simulink model "SimulationEnvManual"  (R2023b)
settings: Solver=VariableStepAuto  StartTime=0.0  StopTime=inf  RelTol=1e-3
undefined symbols (not defined in the file): act_mat, barometer, BIGL, drone, filter, imu, world
libraries: simulink x3, matrix_library x2, aerolibanimutils x2, vrlib x1, sim3dlib x1, uavsim3dlib x1
settings Model: Creator=HP  LastModifiedBy=jelho
settings OptimizationCC: ReuseModelBlockBuffer=off
settings DebuggingCC: AlgebraicLoopMsg=none

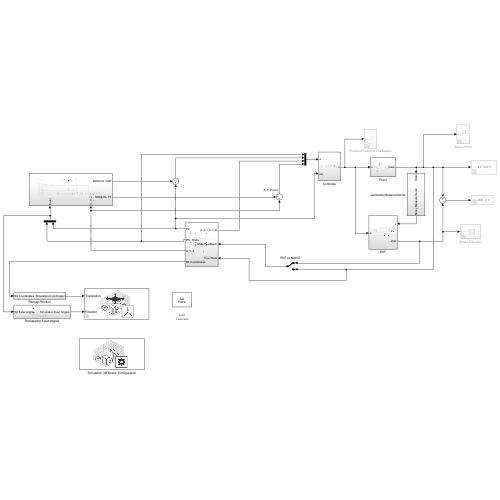
[thumbnail: Simulink's stored preview of the top-level diagram]
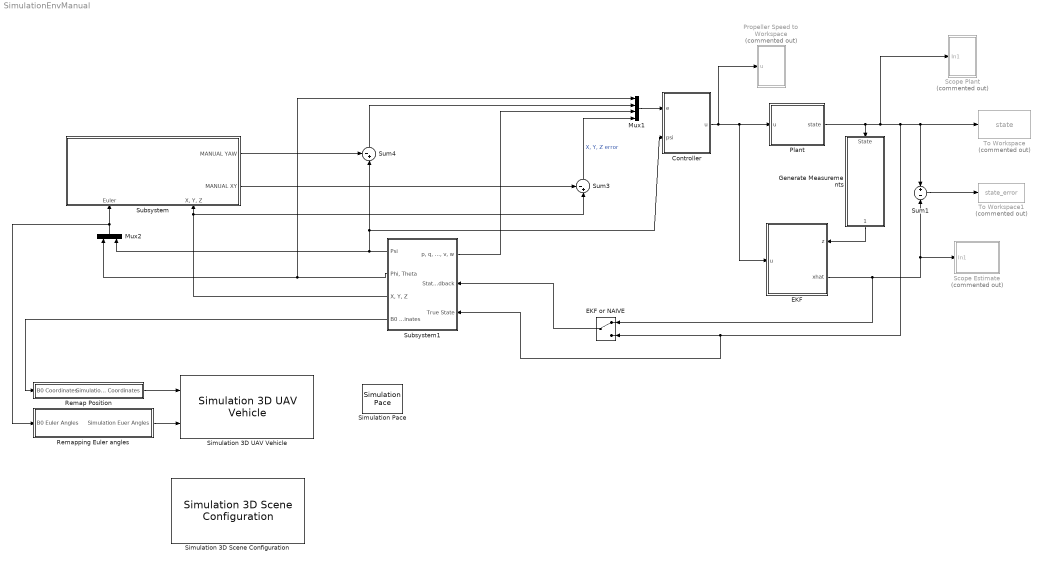
== system SimulationEnvManual ==
  Controller : Subsystem
  EKF : Subsystem
      settings: PortSchema="{\"entries\":[{\"content\":{\"sides\":[{\"content\":{\"connectorIds\":[\"In1\"]},\"type\":\"ConnectorPlacement.EquallySpacedRectSide\",\"uuid\":\"40613573-22c3-4397-8fb4-f3694734863a\"},{\"content\":{\"connectorIds\":[\"In2\",\"Out1\"],\"side\":\"RIGHT\"},\"type\":\"ConnectorPlacement.EquallySpacedRectSide\",\"uuid\":\"0d3695c7-8a5b-4700-a974-c5dffb14488a\"},{\"content\":{\"side\":\"TOP\"},\"type\":\"ConnectorPlacement.EquallySpacedRectSide\",\"uuid\":\"08eac33f-c286-45a0-82f1-214a32c22b76\"},{\"content\":{\"side\":\"BOTTOM\"},\"type\":\"ConnectorPlacement.EquallySpacedRectSide\",\"uuid\":\"51a49a93-d8bc-42ae-9bce-473bc1fc9d07\"}]},\"type\":\"ConnectorPlacement.EquallySpacedConnector\",\"uuid\":\"de3a0f79-73e9-4c25-bf5c-e7b3cc72a00c\"}],\"packageUris\":[\"http://schema.mathworks.com/mf0/Connector/R2020b\"],\"version\":\"1.0\"}"
  EKF or NAIVE : ManualSwitch
  Generate Measurements : Subsystem
  Mux1 : Mux
  Mux2 : Mux  Inputs=2
  Plant : Subsystem
  Propeller Speed to Workspace : Subsystem  Commented=on
  Remap Position : Subsystem
  Remapping Euler angles : Subsystem
  Scope Estimate : Subsystem  Commented=on
  Scope Plant : Subsystem  Commented=on
  Simulation 3D Scene Configuration : sim3dlib/Simulation 3D Scene Configuration  Priority=0  ProjectFormat=Default Scenes  SceneDesc=US city block  ProjectName=C:\Program Files\MATLAB\R2023b\toolbox\shared\sim3d_projects\automotive_project_windows\UE\WindowsNoEditor\VehicleSimulation.exe  ScenePath=/Game/Maps/USCityBlock  EnableOpenDRIVE=off  vehTagList={'Custom';'Scene Origin';'SimulinkVehicle1'}  vehTag=SimulinkVehicle1  FreeCameraInitialTranslation=[0, 0, 0]  FreeCameraDefaultInitialTranslation=[-6, 0, 2]  FreeCameraInitialRotation=[0, 0, 0]  FreeCameraDefaultInitialRotation=[0, -15, 0]  OpVisEn=off  Ts=1/60  EnableWindow=on  EnableRemoteAccess=off  EnableWeather=off  SunAltitude=40.0  SunAzimuth=90  clouds=10  wind=1  fog=0  rain=0  EnableGeospatial=off  OriginHeight=200  OriginLatitude=40.744652  OriginLongitude=-73.988864  MapStyle=Aerial  AdditionalAssetIDs=[]  UseAdvancedSunSky=off  SolarTime=11  TimeZone=-5  Day=21  Month=9  Year=2022  UseDaylightSavingTime=on  DSTStartDay=10  DSTStartMonth=3  DSTEndDay=3  DSTEndMonth=11  DSTSwitchHour=2  sensorTag=MainCamera1  sensorId=1  sensorName=MainCamera1  mountLoc=Origin  offsetFlag=off  tmountOffset=[0, 0, 0]  rmountOffset=[0, 0, 0]  HorizontalResolution=1280  VerticalResolution=720  HorizontalFOV=60  mountPoint=[0 0 0]  mountOrientation=[0 0 0]  aMode=4  ID=1  GeoTrigger=Inactive
      settings: LibrarySourceBlock=uavsim3dlib/Simulation 3D Scene Configuration
  Simulation 3D UAV Vehicle : uavsim3dlib/Simulation 3D UAV Vehicle  Priority=-1  Mesh=Quadrotor  MeshPath=/MathWorksUAVContent/UAVs/HexaRotorUAV/HexaRotor.HexaRotor  Color=Black  ActorName=SimulinkVehicle1  UseGlobalFrame=off  InitialTranslation=[0 0 0]  InitialRotation=[0 0 0]  InitialTranslationGlobal=[0 0 0]  InitialGeoOrigin=[0 0 0]  InitialRotationGlobal=[0 0 0]  SampleTime=-1  ActorType=SimulinkVehicle  ID=1  aMode=4  ActorTag=SimulinkVehicle1
  Simulation Pace : aerolibanimutils/Simulation Pace  SimulationPace=1  SleepMode=Auto  OutputPaceError=off  SampleTime=1/100
  Subsystem : Subsystem
      settings: PortSchema="{\"entries\":[{\"content\":{\"sides\":[{\"content\":{},\"type\":\"ConnectorPlacement.EquallySpacedRectSide\",\"uuid\":\"91d1624f-eb3c-4128-9ca0-0a39a1a4c695\"},{\"content\":{\"connectorIds\":[\"Out1\",\"Out2\"],\"side\":\"RIGHT\"},\"type\":\"ConnectorPlacement.EquallySpacedRectSide\",\"uuid\":\"1eacf8bd-a5e8-4d7e-b2c6-68202da0a464\"},{\"content\":{\"side\":\"TOP\"},\"type\":\"ConnectorPlacement.EquallySpacedRectSide\",\"uuid\":\"881c7496-1eb8-4ab1-ae56-46ea22276703\"},{\"content\":{\"connectorIds\":[\"In1\",\"In2\"],\"side\":\"BOTTOM\"},\"type\":\"ConnectorPlacement.EquallySpacedRectSide\",\"uuid\":\"54f45528-88dd-4514-ad9d-40f26d6e0713\"}]},\"type\":\"ConnectorPlacement.EquallySpacedConnector\",\"uuid\":\"c3aef092-554d-4415-a95e-e2ec15462ee3\"}],\"packageUris\":[\"http://schema.mathworks.com/mf0/Connector/R2020b\"],\"version\":\"1.0\"}"
  Subsystem1 : Subsystem
      settings: PortSchema="{\"entries\":[{\"content\":{\"sides\":[{\"content\":{\"connectorIds\":[\"Out2\",\"Out3\",\"Out4\",\"Out5\"]},\"type\":\"ConnectorPlacement.EquallySpacedRectSide\",\"uuid\":\"a354f8a1-719d-466d-a647-fe8a476dcf5d\"},{\"content\":{\"connectorIds\":[\"Out1\",\"In1\",\"In2\"],\"side\":\"RIGHT\"},\"type\":\"ConnectorPlacement.EquallySpacedRectSide\",\"uuid\":\"b9cb5ede-b59c-409e-8082-fb91c4f2361c\"},{\"content\":{\"side\":\"TOP\"},\"type\":\"ConnectorPlacement.EquallySpacedRectSide\",\"uuid\":\"8ee9585a-2649-44f5-b26b-06d86b499020\"}]},\"type\":\"ConnectorPlacement.EquallySpacedConnector\",\"uuid\":\"6c0311b6-aa0e-4aed-b018-d983f036a7c3\"}],\"packageUris\":[\"http://schema.mathworks.com/mf0/Connector/R2020b\"],\"version\":\"1.0\"}"
  Sum1 : Sum  Inputs=+-
  Sum3 : Sum  Inputs=-+|
  Sum4 : Sum  Inputs=-+|
  To Workspace : ToWorkspace  Commented=on  VariableName=state  SaveFormat=Timeseries  SampleTime=-1
  To Workspace1 : ToWorkspace  Commented=on  VariableName=state_error  SaveFormat=Timeseries  SampleTime=-1
  wires:
  Sum4/1 -> Mux1/2
  Controller/1(u) -> Plant/1(u), EKF/1(u), Propeller Speed to Workspace/1(u)
  Generate Measurements/1(Noisy Measurements) -> EKF/2(z)
  Sum1/1 -> To Workspace1/1
  Plant/1(state) -> Scope Plant/1(In1), Subsystem1/2(True State), EKF or NAIVE/2, To Workspace/1, Sum1/1, Generate Measurements/1(State)
  EKF/1(xhat) -> EKF or NAIVE/1, Sum1/2, Scope Estimate/1(In1)
  Subsystem1/1("p, q, r, u, v, w") -> Mux1/3
  Subsystem/1(MANUAL YAW) -> Sum4/1
  Sum3/1 -> Mux1/4  "X, Y, Z error"
  Subsystem/2(MANUAL XY) -> Sum3/1
  Subsystem1/3("Phi, Theta") -> Mux1/1, Mux2/1
  Subsystem1/2(Psi) -> Mux2/2, Sum4/2, Controller/2(psi)
  Mux2/1 -> Remapping Euler angles/1(B0 Euler Angles), Subsystem/1(Euler)
  Subsystem1/4("X, Y, Z") -> Sum3/2, Subsystem/2("X, Y, Z")
  Remapping Euler angles/1(Simulation Euer Angles) -> Simulation 3D UAV Vehicle/2
  Remap Position/1(Simulation Coordinates) -> Simulation 3D UAV Vehicle/1
  Mux1/1 -> Controller/1(e)
  EKF or NAIVE/1 -> Subsystem1/1(State Feedback)
  Subsystem1/5(B0 Coordinates) -> Remap Position/1(B0 Coordinates)

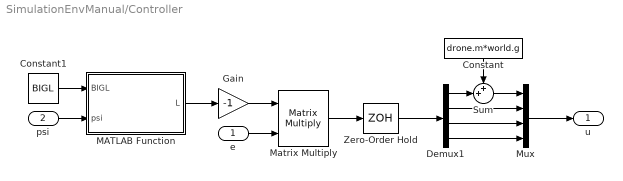
== system SimulationEnvManual/Controller ==
  e : Inport
  psi : Inport  Port=2
  Constant : Constant  Value=drone.m*world.g
  Constant1 : Constant  Value=BIGL
  Demux1 : Demux
  Gain : Gain  Gain=-1
  MATLAB Function : MATLAB Function  TreatAsAtomicUnit=on
  Matrix Multiply : Product  Multiplication=Matrix(*)
  Mux : Mux
  Sum : Sum  Inputs=++|
  Zero-Order Hold : ZeroOrderHold  SampleTime=0.01
  u : Outport
  wires:
  Demux1/3 -> Mux/3
  Demux1/2 -> Mux/2
  Mux/1 -> u/1
  Demux1/4 -> Mux/4
  Demux1/1 -> Sum/2
  Sum/1 -> Mux/1
  Constant/1 -> Sum/1
  Zero-Order Hold/1 -> Demux1/1
  e/1 -> Matrix Multiply/2
  Gain/1 -> Matrix Multiply/1
  Matrix Multiply/1 -> Zero-Order Hold/1
  MATLAB Function/1(L) -> Gain/1
  Constant1/1 -> MATLAB Function/1(BIGL)
  psi/1 -> MATLAB Function/2(psi)

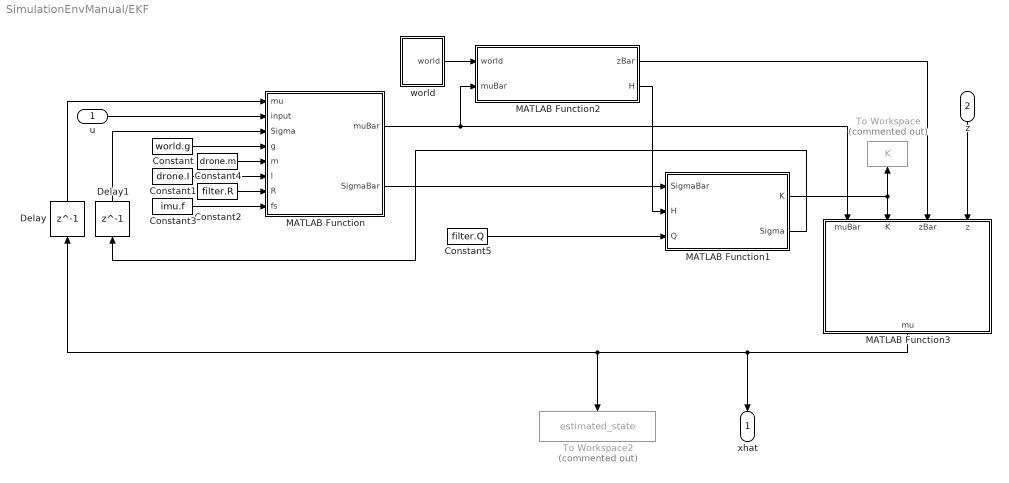
== system SimulationEnvManual/EKF ==
  u : Inport
  z : Inport  Port=2
  Constant : Constant  Value=world.g
  Constant1 : Constant  Value=drone.I
  Constant2 : Constant  Value=filter.R
  Constant3 : Constant  Value=imu.f
  Constant4 : Constant  Value=drone.m
  Constant5 : Constant  Value=filter.Q
  Delay : Delay  DelayLength=1  InitialCondition=filter.mu_0  SampleTime=0.01
  Delay1 : Delay  DelayLength=1  InitialCondition=filter.Sigma_0  SampleTime=0.01
  MATLAB Function : MATLAB Function  TreatAsAtomicUnit=on
  MATLAB Function1 : MATLAB Function  TreatAsAtomicUnit=on
  MATLAB Function2 : MATLAB Function  TreatAsAtomicUnit=on
  MATLAB Function3 : MATLAB Function  TreatAsAtomicUnit=on
  To Workspace : ToWorkspace  Commented=on  VariableName=K  SampleTime=-1
  To Workspace2 : ToWorkspace  Commented=on  VariableName=estimated_state  SaveFormat=Timeseries  SampleTime=-1
  world : Subsystem
  xhat : Outport
  wires:
  Constant2/1 -> MATLAB Function/7(R)
  MATLAB Function3/1(mu) -> Delay/1, To Workspace2/1, xhat/1
  MATLAB Function1/2(Sigma) -> Delay1/1
  MATLAB Function/1(muBar) -> MATLAB Function3/1(muBar), MATLAB Function2/2(muBar)
  Constant/1 -> MATLAB Function/4(g)
  MATLAB Function2/2(H) -> MATLAB Function1/2(H)
  Delay/1 -> MATLAB Function/1(mu)
  Constant1/1 -> MATLAB Function/6(I)
  MATLAB Function1/1(K) -> MATLAB Function3/2(K), To Workspace/1
  Constant5/1 -> MATLAB Function1/3(Q)
  MATLAB Function2/1(zBar) -> MATLAB Function3/3(zBar)
  Delay1/1 -> MATLAB Function/3(Sigma)
  Constant3/1 -> MATLAB Function/8(fs)
  Constant4/1 -> MATLAB Function/5(m)
  z/1 -> MATLAB Function3/4(z)
  MATLAB Function/2(SigmaBar) -> MATLAB Function1/1(SigmaBar)
  u/1 -> MATLAB Function/2(input)
  world/1(world) -> MATLAB Function2/1(world)

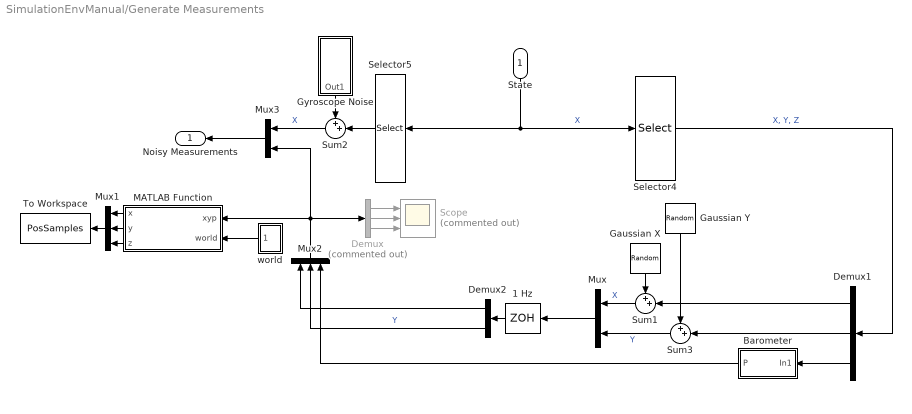
== system SimulationEnvManual/Generate Measurements ==
  State : Inport
  1 Hz : ZeroOrderHold
  Barometer : Subsystem
  Demux : Demux  Commented=on  Outputs=3
  Demux1 : Demux  Outputs=3
  Demux2 : Demux  Outputs=2
  Gaussian X : RandomNumber  Variance=4  Seed=[43121]  SampleTime=0.1
  Gaussian Y : RandomNumber  Variance=4  Seed=[43341]  SampleTime=0.1
  Gyroscope Noise : Subsystem
  MATLAB Function : MATLAB Function  TreatAsAtomicUnit=on
  Mux : Mux  Inputs=2
  Mux1 : Mux  Inputs=3
  Mux2 : Mux  Inputs=3
  Mux3 : Mux  Inputs=2
  Scope : Scope  Commented=on  NumInputPorts=3
  Selector4 : Selector  InputPortWidth=12  IndexOptions=Index vector (dialog)  Indices=[10 11 12]  OutputSizes=1
  Selector5 : Selector  InputPortWidth=12  IndexOptions=Index vector (dialog)  Indices=[1 2 3 4 5 6]  OutputSizes=1
  Sum1 : Sum  Inputs=++|
  Sum2 : Sum  Inputs=++|
  Sum3 : Sum  Inputs=++|
  To Workspace : ToWorkspace  VariableName=PosSamples  SaveFormat=Timeseries  SampleTime=-1
  world : Subsystem
  Noisy Measurements : Outport
  wires:
  Selector4/1 -> Demux1/1  "X, Y, Z"
  Mux2/1 -> Demux/1, Mux3/2, MATLAB Function/1(xyp)
  Demux2/1 -> Mux2/1
  1 Hz/1 -> Demux2/1
  Mux3/1 -> Noisy Measurements/1
  Mux/1 -> 1 Hz/1
  Demux2/2 -> Mux2/2  "Y"
  Gaussian X/1 -> Sum1/1
  Sum1/1 -> Mux/1  "X"
  Demux1/1 -> Sum1/2
  Sum3/1 -> Mux/2  "Y"
  Demux1/2 -> Sum3/2
  Gaussian Y/1 -> Sum3/1
  Demux/1 -> Scope/1
  Demux/2 -> Scope/2
  Demux/3 -> Scope/3
  Demux1/3 -> Barometer/1(In1)
  world/1(Out1) -> MATLAB Function/2(world)
  MATLAB Function/2(y) -> Mux1/2
  MATLAB Function/1(x) -> Mux1/1
  MATLAB Function/3(z) -> Mux1/3
  Mux1/1 -> To Workspace/1
  Selector5/1 -> Sum2/2
  Sum2/1 -> Mux3/1  "X"
  Gyroscope Noise/1(Out1) -> Sum2/1
  State/1 -> Selector5/1, Selector4/1  "X"
  Barometer/1(P) -> Mux2/3

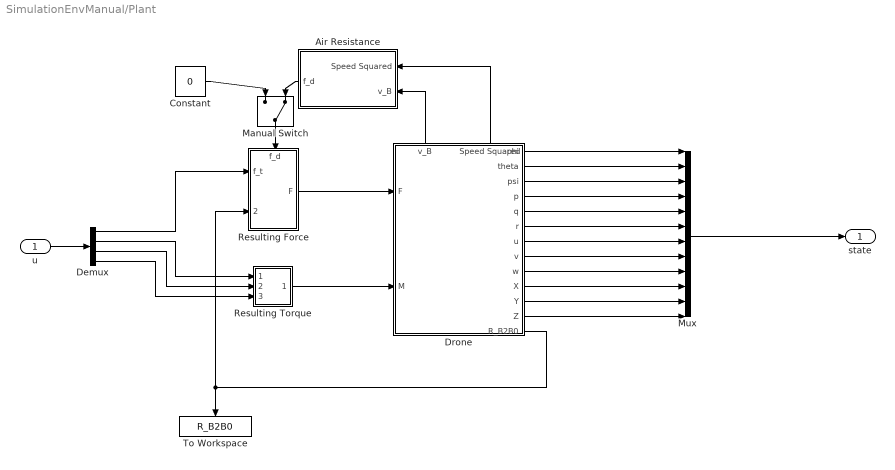
== system SimulationEnvManual/Plant ==
  u : Inport
  Air Resistance : Subsystem
  Constant : Constant  Value=0
  Demux : Demux
  Drone : Subsystem
      settings: PortSchema="{\"entries\":[{\"content\":{\"sides\":[{\"content\":{\"connectorIds\":[\"In1\",\"In2\"]},\"type\":\"ConnectorPlacement.EquallySpacedRectSide\",\"uuid\":\"8ffad7a2-32ec-43eb-87ee-fb2abc5db72d\"},{\"content\":{\"connectorIds\":[\"Out1\",\"Out2\",\"Out3\",\"Out4\",\"Out5\",\"Out6\",\"Out7\",\"Out8\",\"Out9\",\"Out10\",\"Out11\",\"Out12\",\"Out13\"],\"side\":\"RIGHT\"},\"type\":\"ConnectorPlacement.EquallySpacedRectSide\",\"uuid\":\"ca8d09d3-eea8-43a3-a12c-d896baab46a4\"},{\"content\":{\"connectorIds\":[\"Out14\",\"Out15\"],\"side\":\"TOP\"},\"type\":\"ConnectorPlacement.EquallySpacedRectSide\",\"uuid\":\"dfab79fc-8469-4116-b735-45bfaccfab37\"}]},\"type\":\"ConnectorPlacement.EquallySpacedConnector\",\"uuid\":\"bfc700f2-23fb-440c-b21c-b50295174d97\"}],\"packageUris\":[\"http://schema.mathworks.com/mf0/Connector/R2020b\"],\"version\":\"1.0\"}"
  Manual Switch : ManualSwitch  CurrentSetting=0
  Mux : Mux  Inputs=12
  Resulting Force : Subsystem
      settings: PortSchema="{\"entries\":[{\"content\":{\"sides\":[{\"content\":{\"connectorIds\":[\"In1\",\"In2\"]},\"type\":\"ConnectorPlacement.EquallySpacedRectSide\",\"uuid\":\"15f6bfea-ca78-407b-a070-46266de37f17\"},{\"content\":{\"connectorIds\":[\"Out1\"],\"side\":\"RIGHT\"},\"type\":\"ConnectorPlacement.EquallySpacedRectSide\",\"uuid\":\"1ac3e3a8-f699-47b6-93e9-6e96eb41779e\"},{\"content\":{\"connectorIds\":[\"In3\"],\"side\":\"TOP\"},\"type\":\"ConnectorPlacement.EquallySpacedRectSide\",\"uuid\":\"5f280c1d-1924-4695-afed-fbf3b3e218ac\"}]},\"type\":\"ConnectorPlacement.EquallySpacedConnector\",\"uuid\":\"fee2f4d4-3ff7-4dd2-b01a-205ded0d46ee\"}],\"packageUris\":[\"http://schema.mathworks.com/mf0/Connector/R2020b\"],\"version\":\"1.0\"}"
  Resulting Torque : Subsystem
  To Workspace : ToWorkspace  VariableName=R_B2B0  SampleTime=-1
  state : Outport
  wires:
  Drone/7(u) -> Mux/7
  Drone/2(theta) -> Mux/2
  Drone/4(p) -> Mux/4
  Drone/1(phi) -> Mux/1
  Drone/6(r) -> Mux/6
  Drone/9(w) -> Mux/9
  Resulting Torque/1(Out1) -> Drone/2(M)
  Drone/5(q) -> Mux/5
  Resulting Force/1(F) -> Drone/1(F)
  Drone/3(psi) -> Mux/3
  Drone/11(Y) -> Mux/11
  Drone/10(X) -> Mux/10
  Drone/8(v) -> Mux/8
  Drone/12(Z) -> Mux/12
  Drone/13(R_B2B0) -> Resulting Force/2(R_B2B0), To Workspace/1
  u/1 -> Demux/1
  Drone/14(v_B) -> Air Resistance/2(v_B)
  Drone/15(Speed Squared) -> Air Resistance/1(Speed Squared)
  Demux/1 -> Resulting Force/1(f_t)
  Demux/2 -> Resulting Torque/1(tau_x)
  Demux/3 -> Resulting Torque/2(tau_y)
  Demux/4 -> Resulting Torque/3(tau_z)
  Mux/1 -> state/1
  Manual Switch/1 -> Resulting Force/3(f_d)
  Air Resistance/1(f_d) -> Manual Switch/2
  Constant/1 -> Manual Switch/1

== system SimulationEnvManual/Propeller Speed to Workspace ==
  u : Inport
  Constant1 : Constant  Value=act_mat
  Matrix Multiply : Product  Multiplication=Matrix(*)
  To Workspace1 : ToWorkspace  VariableName=Input  SaveFormat=Timeseries  SampleTime=-1
  To Workspace2 : ToWorkspace  VariableName=PropSpeed  SaveFormat=Timeseries  SampleTime=-1
  wires:
  Matrix Multiply/1 -> To Workspace2/1
  u/1 -> Matrix Multiply/2, To Workspace1/1
  Constant1/1 -> Matrix Multiply/1

== system SimulationEnvManual/Remap Position ==
  B0 Coordinates : Inport
  Demux : Demux  Outputs=3
  Gain : Gain  Gain=-1
  Mux4 : Mux  Inputs=3
  Simulation Coordinates : Outport
  wires:
  Gain/1 -> Mux4/3
  Demux/1 -> Mux4/1
  B0 Coordinates/1 -> Demux/1
  Demux/3 -> Gain/1
  Mux4/1 -> Simulation Coordinates/1
  Demux/2 -> Mux4/2

== system SimulationEnvManual/Remapping Euler angles ==
  B0 Euler Angles : Inport
  Demux : Demux  Outputs=3
  Gain1 : Gain  Gain=-1
  Gain2 : Gain  Gain=-1
  Mux4 : Mux  Inputs=3
  Simulation Euer Angles : Outport
  wires:
  Demux/1 -> Gain2/1  "Roll"
  Demux/3 -> Mux4/1  "Yaw"
  Mux4/1 -> Simulation Euer Angles/1
  Demux/2 -> Gain1/1  "Pitch"
  B0 Euler Angles/1 -> Demux/1
  Gain1/1 -> Mux4/2
  Gain2/1 -> Mux4/3

== system SimulationEnvManual/Scope Estimate ==
  In1 : Inport
  Demux1 : Demux  Outputs=12
  Scope2 : Scope  NumInputPorts=12
  wires:
  Demux1/3 -> Scope2/3  "psi"
  Demux1/9 -> Scope2/9  "w"
  Demux1/10 -> Scope2/10  "X"
  Demux1/8 -> Scope2/8  "v"
  Demux1/5 -> Scope2/5  "q"
  Demux1/2 -> Scope2/2  "theta"
  Demux1/12 -> Scope2/12  "Z"
  Demux1/4 -> Scope2/4  "p"
  Demux1/6 -> Scope2/6  "r"
  Demux1/11 -> Scope2/11  "Y"
  Demux1/7 -> Scope2/7  "u"
  Demux1/1 -> Scope2/1  "phi"
  In1/1 -> Demux1/1

== system SimulationEnvManual/Scope Plant ==
  In1 : Inport
  Demux : Demux  Outputs=12
  Scope : Scope  NumInputPorts=12
  wires:
  Demux/9 -> Scope/9  "w"
  Demux/4 -> Scope/4  "p"
  Demux/12 -> Scope/12  "Z"
  Demux/2 -> Scope/2  "theta"
  Demux/6 -> Scope/6  "r"
  Demux/1 -> Scope/1  "phi"
  Demux/11 -> Scope/11  "Y"
  Demux/7 -> Scope/7  "u"
  Demux/10 -> Scope/10  "X"
  Demux/8 -> Scope/8  "v"
  Demux/3 -> Scope/3  "psi"
  Demux/5 -> Scope/5  "q"
  In1/1 -> Demux/1

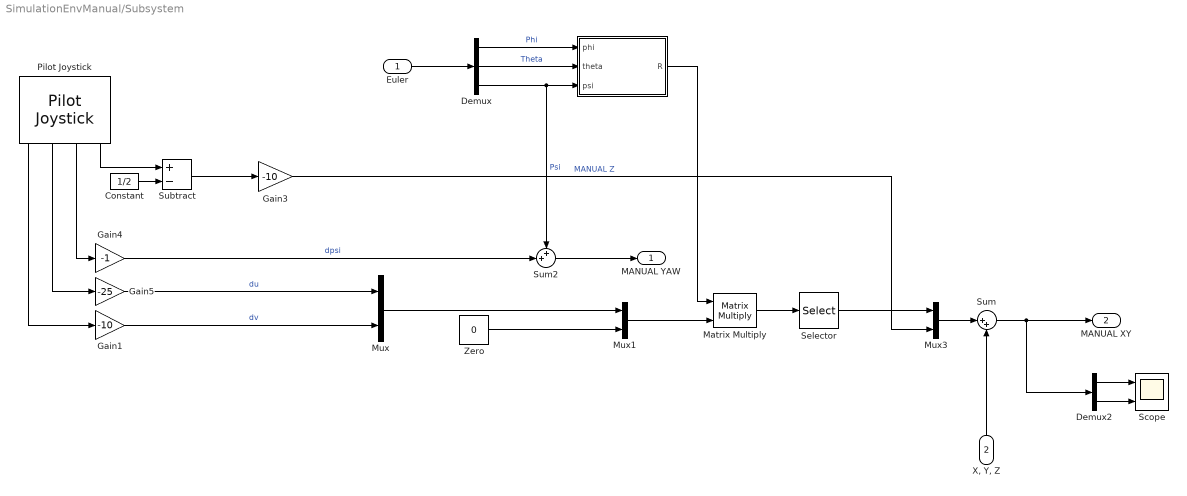
== system SimulationEnvManual/Subsystem ==
  Euler : Inport
  "X, Y, Z" : Inport  Port=2
  " " : MATLAB Function  TreatAsAtomicUnit=on
  Constant : Constant  Value=1/2
  Demux : Demux  Outputs=3
  Demux2 : Demux  Outputs=2
  Gain1 : Gain  Gain=-10
  Gain3 : Gain  Gain=-10
  Gain4 : Gain  Gain=-1
  Gain5 : Gain  Gain=-25
  Matrix Multiply : Product  Multiplication=Matrix(*)
  Mux : Mux  Inputs=2
  Mux1 : Mux  Inputs=2
  Mux3 : Mux  Inputs=2
  Pilot Joystick : aerolibanimutils/Pilot Joystick  JoystickID=Joystick1  OutputConfiguration=FourAxis  SampleTime=1/30
  Scope : Scope  NumInputPorts=2
  Selector : Selector  InputPortWidth=3  IndexOptions=Index vector (dialog)  Indices=[1 2]  OutputSizes=1
  Subtract : Sum  Inputs=+-
  Sum : Sum  Inputs=|++
  Sum2 : Sum  Inputs=++|
  Zero : Constant  Value=0  OutDataTypeStr=Inherit: Inherit via back propagation
  MANUAL YAW : Outport
  MANUAL XY : Outport  Port=2
  wires:
  Pilot Joystick/2 -> Gain5/1
  Pilot Joystick/3 -> Gain4/1
  Gain4/1 -> Sum2/2  "dpsi"
  Pilot Joystick/1 -> Gain1/1
  Pilot Joystick/4 -> Subtract/1
  Constant/1 -> Subtract/2
  Subtract/1 -> Gain3/1
  Gain3/1 -> Mux3/2  "MANUAL Z"
  Mux/1 -> Mux1/1
  Gain5/1 -> Mux/1  "du"
  Gain1/1 -> Mux/2  "dv"
  Euler/1 -> Demux/1
  Demux/1 -> " "/1(phi)  "Phi"
  Demux/2 -> " "/2(theta)  "Theta"
  Demux/3 -> " "/3(psi), Sum2/1  "Psi"
  Zero/1 -> Mux1/2
  Mux1/1 -> Matrix Multiply/2
  " "/1(R) -> Matrix Multiply/1
  Matrix Multiply/1 -> Selector/1
  Selector/1 -> Mux3/1
  "X, Y, Z"/1 -> Sum/2
  Sum/1 -> MANUAL XY/1, Demux2/1
  Sum2/1 -> MANUAL YAW/1
  Demux2/1 -> Scope/1
  Demux2/2 -> Scope/2
  Mux3/1 -> Sum/1

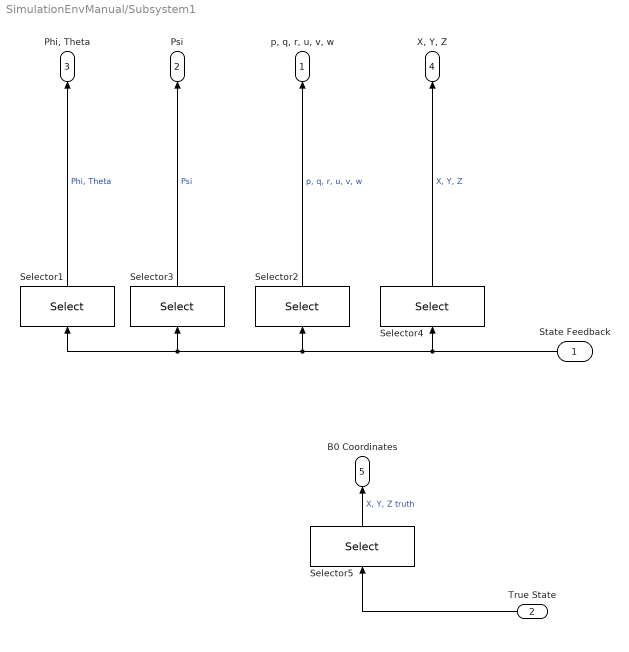
== system SimulationEnvManual/Subsystem1 ==
  State Feedback : Inport
  True State : Inport  Port=2
  Selector1 : Selector  InputPortWidth=12  IndexOptions=Index vector (dialog)  Indices=[1 2]  OutputSizes=1
  Selector2 : Selector  InputPortWidth=12  IndexOptions=Index vector (dialog)  Indices=[4 5 6 7 8 9]  OutputSizes=1
  Selector3 : Selector  InputPortWidth=12  IndexOptions=Index vector (dialog)  Indices=[3]  OutputSizes=1
  Selector4 : Selector  InputPortWidth=12  IndexOptions=Index vector (dialog)  Indices=[10 11 12]  OutputSizes=1
  Selector5 : Selector  InputPortWidth=12  IndexOptions=Index vector (dialog)  Indices=[10 11 12]  OutputSizes=1
  "p, q, r, u, v, w" : Outport
  Psi : Outport  Port=2
  "Phi, Theta" : Outport  Port=3
  "X, Y, Z" : Outport  Port=4
  B0 Coordinates : Outport  Port=5
  wires:
  Selector3/1 -> Psi/1  "Psi"
  Selector4/1 -> "X, Y, Z"/1  "X, Y, Z"
  State Feedback/1 -> Selector4/1, Selector1/1, Selector3/1, Selector2/1
  Selector1/1 -> "Phi, Theta"/1  "Phi, Theta"
  Selector2/1 -> "p, q, r, u, v, w"/1  "p, q, r, u, v, w"
  True State/1 -> Selector5/1
  Selector5/1 -> B0 Coordinates/1  "X, Y, Z truth"

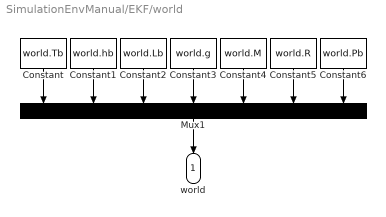
== system SimulationEnvManual/EKF/world ==
  Constant : Constant  Value=world.Tb
  Constant1 : Constant  Value=world.hb
  Constant2 : Constant  Value=world.Lb
  Constant3 : Constant  Value=world.g
  Constant4 : Constant  Value=world.M
  Constant5 : Constant  Value=world.R
  Constant6 : Constant  Value=world.Pb
  Mux1 : Mux  Inputs=7
  world : Outport
  wires:
  Constant2/1 -> Mux1/3
  Mux1/1 -> world/1
  Constant4/1 -> Mux1/5
  Constant3/1 -> Mux1/4
  Constant5/1 -> Mux1/6
  Constant/1 -> Mux1/1
  Constant1/1 -> Mux1/2
  Constant6/1 -> Mux1/7

== system SimulationEnvManual/Generate Measurements/Barometer ==
  In1 : Inport
  10 Hz : ZeroOrderHold  SampleTime=0.1
  Constant : Constant  Value=barometer.std
  MATLAB Function : MATLAB Function  TreatAsAtomicUnit=on
  world : Subsystem
  P : Outport
  wires:
  In1/1 -> 10 Hz/1
  10 Hz/1 -> MATLAB Function/1(Z)
  Constant/1 -> MATLAB Function/2(std)
  MATLAB Function/1(P) -> P/1  "P"
  world/1(Out1) -> MATLAB Function/3(world)

== system SimulationEnvManual/Generate Measurements/Gyroscope Noise ==
  " Phi" : RandomNumber  Variance=[((pi/180))^2]  Seed=[43341]  SampleTime=0.01
  " Psi" : RandomNumber  Variance=[((pi/180))^2]  Seed=[43751]  SampleTime=0.01
  " Theta" : RandomNumber  Variance=[((pi/180))^2]  Seed=[47341]  SampleTime=0.01
  " p" : RandomNumber  Variance=[((pi/180)*2.5)^2]  Seed=[41341]  SampleTime=0.01
  " q" : RandomNumber  Variance=[((pi/180)*2.5)^2]  Seed=[43631]  SampleTime=0.01
  " r" : RandomNumber  Variance=[((pi/180)*2.5)^2]  Seed=[67842]  SampleTime=0.01
  Mux4 : Mux  Inputs=6
  Out1 : Outport
  wires:
  " r"/1 -> Mux4/6
  " q"/1 -> Mux4/5
  Mux4/1 -> Out1/1
  " p"/1 -> Mux4/4
  " Phi"/1 -> Mux4/1
  " Theta"/1 -> Mux4/2
  " Psi"/1 -> Mux4/3

== system SimulationEnvManual/Generate Measurements/world ==
  Constant : Constant  Value=world.Tb
  Constant1 : Constant  Value=world.hb
  Constant2 : Constant  Value=world.Lb
  Constant3 : Constant  Value=world.g
  Constant4 : Constant  Value=world.M
  Constant5 : Constant  Value=world.R
  Constant6 : Constant  Value=world.Pb
  Mux1 : Mux  Inputs=7
  Out1 : Outport
  wires:
  Constant2/1 -> Mux1/3
  Mux1/1 -> Out1/1
  Constant4/1 -> Mux1/5
  Constant3/1 -> Mux1/4
  Constant5/1 -> Mux1/6
  Constant/1 -> Mux1/1
  Constant1/1 -> Mux1/2
  Constant6/1 -> Mux1/7

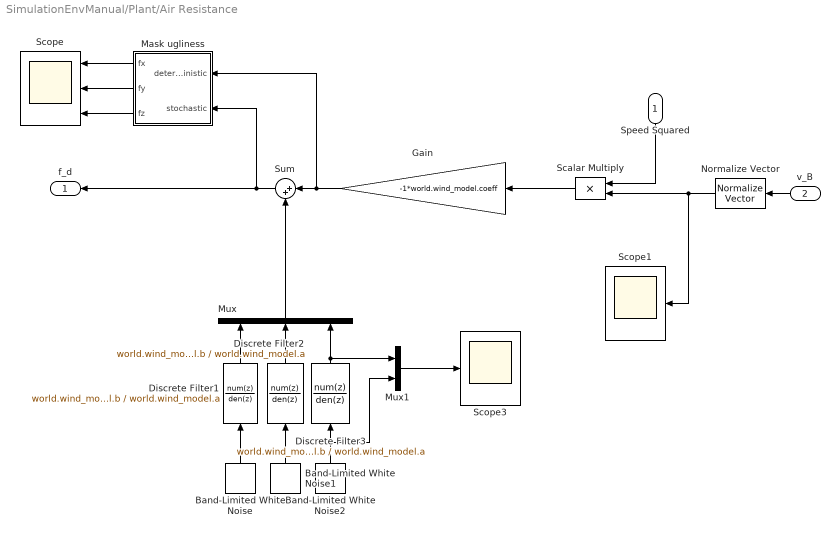
== system SimulationEnvManual/Plant/Air Resistance ==
  Speed Squared : Inport
  v_B : Inport  Port=2
  Band-Limited White Noise : simulink/Sources/Band-Limited White Noise  Cov=[0.001]  Ts=0.01  seed=[23351]
  Band-Limited White Noise1 : simulink/Sources/Band-Limited White Noise  Cov=[0.001]  Ts=0.01  seed=[23341]
  Band-Limited White Noise2 : simulink/Sources/Band-Limited White Noise  Cov=[0.001]  Ts=0.01  seed=[86328]
  Discrete Filter1 : DiscreteFilter  Numerator=world.wind_model.b  Denominator=world.wind_model.a
  Discrete Filter2 : DiscreteFilter  Numerator=world.wind_model.b  Denominator=world.wind_model.a
  Discrete Filter3 : DiscreteFilter  Numerator=world.wind_model.b  Denominator=world.wind_model.a
  Gain : Gain  Gain=-1*world.wind_model.coeff
  Mask ugliness : Subsystem
  Mux : Mux  Inputs=3
  Mux1 : Mux  Inputs=2
  Normalize Vector : vrlib/Utilities/Normalize Vector  maxzero=0
  Scalar Multiply : Product
  Scope : Scope  NumInputPorts=3
  Scope1 : Scope
  Scope3 : Scope
  Sum : Sum  Inputs=|++
  f_d : Outport
  wires:
  Normalize Vector/1 -> Scope1/1, Scalar Multiply/2
  Band-Limited White Noise/1 -> Discrete Filter1/1
  Band-Limited White Noise2/1 -> Mux1/2, Discrete Filter3/1
  Mux/1 -> Sum/2
  Gain/1 -> Mask ugliness/1(deterministic), Sum/1
  Sum/1 -> Mask ugliness/2(stochastic), f_d/1
  Mask ugliness/1(fx) -> Scope/1
  Mask ugliness/2(fy) -> Scope/2
  Mask ugliness/3(fz) -> Scope/3
  Discrete Filter1/1 -> Mux/1
  Discrete Filter2/1 -> Mux/2
  Discrete Filter3/1 -> Mux/3, Mux1/1
  v_B/1 -> Normalize Vector/1
  Scalar Multiply/1 -> Gain/1
  Speed Squared/1 -> Scalar Multiply/1
  Mux1/1 -> Scope3/1
  Band-Limited White Noise1/1 -> Discrete Filter2/1

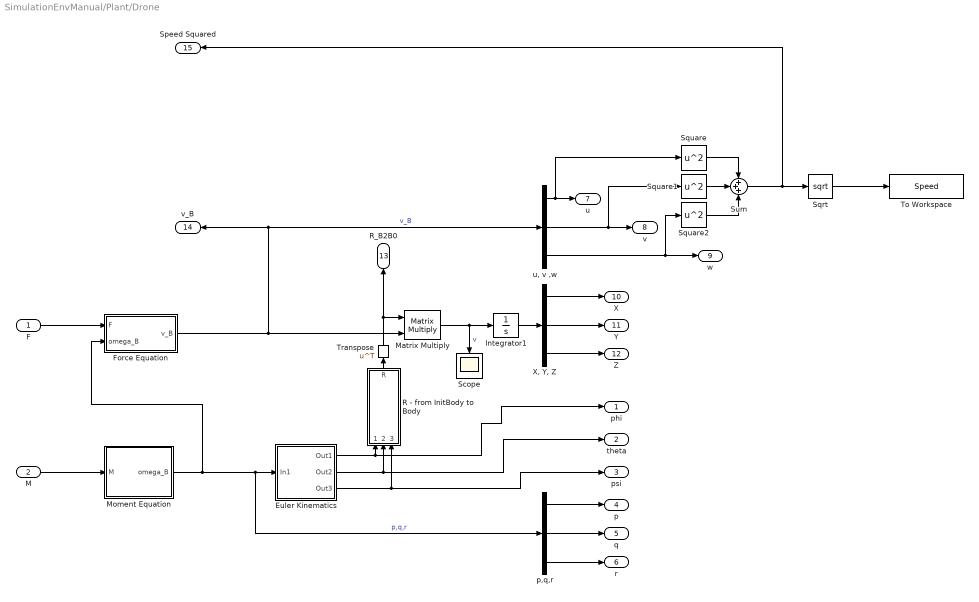
== system SimulationEnvManual/Plant/Drone ==
  F : Inport
  M : Inport  Port=2
  Euler Kinematics : Subsystem
  Force Equation : Subsystem
  Integrator1 : Integrator  InitialCondition=[0,0,0]
  Matrix Multiply : Product  Multiplication=Matrix(*)
  Moment Equation : Subsystem
  R - from InitBody to Body : MATLAB Function  TreatAsAtomicUnit=on
  Scope : Scope
  Sqrt : Sqrt
  Square : Math  Operator=square
  Square1 : Math  Operator=square
  Square2 : Math  Operator=square
  Sum : Sum  Inputs=+++
  To Workspace : ToWorkspace  VariableName=Speed  SaveFormat=Timeseries  SampleTime=-1
  Transpose : Math  Operator=transpose
  "X, Y, Z" : Demux  Outputs=3
  p,q,r : Demux  Outputs=3
  "u, v ,w" : Demux  Outputs=3
  phi : Outport
  theta : Outport  Port=2
  psi : Outport  Port=3
  p : Outport  Port=4
  q : Outport  Port=5
  r : Outport  Port=6
  u : Outport  Port=7
  v : Outport  Port=8
  w : Outport  Port=9
  X : Outport  Port=10
  Y : Outport  Port=11
  Z : Outport  Port=12
  R_B2B0 : Outport  Port=13
  v_B : Outport  Port=14
  Speed Squared : Outport  Port=15
  wires:
  Force Equation/1(v_B) -> Matrix Multiply/2, "u, v ,w"/1, v_B/1  "v_B"
  Euler Kinematics/2(Out2) -> R - from InitBody to Body/2(theta), theta/1
  Euler Kinematics/3(Out3) -> psi/1, R - from InitBody to Body/3(psi)
  "u, v ,w"/2 -> Square1/1, v/1
  "X, Y, Z"/1 -> X/1
  Integrator1/1 -> "X, Y, Z"/1
  Moment Equation/1(omega_B) -> p,q,r/1, Euler Kinematics/1(In1), Force Equation/2(omega_B)  "p,q,r"
  Euler Kinematics/1(Out1) -> R - from InitBody to Body/1(phi), phi/1
  "X, Y, Z"/2 -> Y/1
  Matrix Multiply/1 -> Integrator1/1, Scope/1  "v"
  F/1 -> Force Equation/1(F)
  "X, Y, Z"/3 -> Z/1
  M/1 -> Moment Equation/1(M)
  "u, v ,w"/3 -> Square2/1, w/1
  "u, v ,w"/1 -> Square/1, u/1
  p,q,r/2 -> q/1
  p,q,r/1 -> p/1
  p,q,r/3 -> r/1
  R - from InitBody to Body/1(R) -> Transpose/1
  Transpose/1 -> Matrix Multiply/1, R_B2B0/1
  Square/1 -> Sum/1
  Square1/1 -> Sum/2
  Square2/1 -> Sum/3
  Sum/1 -> Speed Squared/1, Sqrt/1
  Sqrt/1 -> To Workspace/1

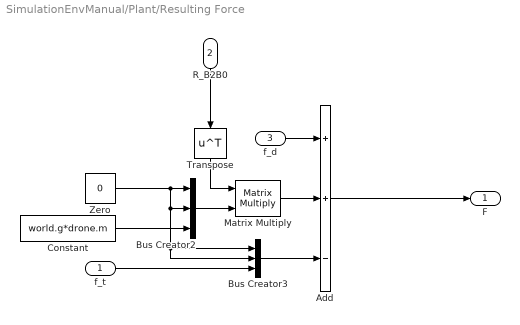
== system SimulationEnvManual/Plant/Resulting Force ==
  f_t : Inport
  R_B2B0 : Inport  Port=2
  f_d : Inport  Port=3
  Add : Sum  Inputs=++-
  Bus Creator2 : BusCreator  Inputs=3
  Bus Creator3 : BusCreator  Inputs=3
  Constant : Constant  Value=world.g*drone.m
  Matrix Multiply : Product  Multiplication=Matrix(*)
  Transpose : Math  Operator=transpose
  Zero : Constant  Value=0  OutDataTypeStr=Inherit: Inherit via back propagation
  F : Outport
  wires:
  Matrix Multiply/1 -> Add/2
  Bus Creator2/1 -> Matrix Multiply/2
  Add/1 -> F/1
  Zero/1 -> Bus Creator2/2, Bus Creator3/1, Bus Creator3/2, Bus Creator2/1
  R_B2B0/1 -> Transpose/1
  Constant/1 -> Bus Creator2/3
  Transpose/1 -> Matrix Multiply/1
  f_t/1 -> Bus Creator3/3
  Bus Creator3/1 -> Add/3
  f_d/1 -> Add/1

== system SimulationEnvManual/Plant/Resulting Torque ==
  tau_x : Inport
  tau_y : Inport  Port=2
  tau_z : Inport  Port=3
  Bus Creator2 : BusCreator  Inputs=3
  Out1 : Outport
  wires:
  tau_z/1 -> Bus Creator2/3
  Bus Creator2/1 -> Out1/1
  tau_x/1 -> Bus Creator2/1
  tau_y/1 -> Bus Creator2/2

== system SimulationEnvManual/Generate Measurements/Barometer/world ==
  Constant : Constant  Value=world.Tb
  Constant1 : Constant  Value=world.hb
  Constant2 : Constant  Value=world.Lb
  Constant3 : Constant  Value=world.g
  Constant4 : Constant  Value=world.M
  Constant5 : Constant  Value=world.R
  Constant6 : Constant  Value=world.Pb
  Mux1 : Mux  Inputs=7
  Out1 : Outport
  wires:
  Constant2/1 -> Mux1/3
  Mux1/1 -> Out1/1
  Constant4/1 -> Mux1/5
  Constant3/1 -> Mux1/4
  Constant5/1 -> Mux1/6
  Constant/1 -> Mux1/1
  Constant1/1 -> Mux1/2
  Constant6/1 -> Mux1/7

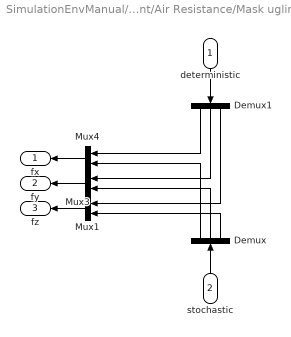
== system SimulationEnvManual/Plant/Air Resistance/Mask ugliness ==
  deterministic : Inport
  stochastic : Inport  Port=2
  Demux : Demux  Outputs=3
  Demux1 : Demux  Outputs=3
  Mux1 : Mux  Inputs=2
  Mux3 : Mux  Inputs=2
  Mux4 : Mux  Inputs=2
  fx : Outport
  fy : Outport  Port=2
  fz : Outport  Port=3
  wires:
  Mux1/1 -> fz/1
  Mux3/1 -> fy/1
  Mux4/1 -> fx/1
  stochastic/1 -> Demux/1
  Demux/1 -> Mux4/2
  Demux/2 -> Mux3/2
  Demux/3 -> Mux1/2
  deterministic/1 -> Demux1/1
  Demux1/1 -> Mux4/1
  Demux1/2 -> Mux3/1
  Demux1/3 -> Mux1/1

== system SimulationEnvManual/Plant/Drone/Euler Kinematics ==
  In1 : Inport
  Integrator3 : Integrator  InitialCondition=imu.Euler0
  MATLAB Function : MATLAB Function  TreatAsAtomicUnit=on
  "p, q, r" : Demux  Outputs=3
  "phi, theta, psi" : Demux  Outputs=3
  Out1 : Outport
  Out2 : Outport  Port=2
  Out3 : Outport  Port=3
  wires:
  Integrator3/1 -> "phi, theta, psi"/1
  "p, q, r"/3 -> MATLAB Function/3(r)
  "phi, theta, psi"/2 -> Out2/1, MATLAB Function/5(theta)
  In1/1 -> "p, q, r"/1
  MATLAB Function/1(omega) -> Integrator3/1  "omega"
  "p, q, r"/2 -> MATLAB Function/2(q)
  "phi, theta, psi"/1 -> Out1/1, MATLAB Function/4(phi)
  "p, q, r"/1 -> MATLAB Function/1(p)
  "phi, theta, psi"/3 -> Out3/1

== system SimulationEnvManual/Plant/Drone/Force Equation ==
  F : Inport
  omega_B : Inport  Port=2
  Cross Product : matrix_library/Cross Product
  Integrator : Integrator
  Multiply : Gain  Gain=1/drone.m
  Sum : Sum  Inputs=+-
  v_B : Outport
  wires:
  Sum/1 -> Integrator/1  "v_BDot"
  Cross Product/1 -> Sum/2
  Integrator/1 -> v_B/1, Cross Product/2  "v_B"
  Multiply/1 -> Sum/1
  F/1 -> Multiply/1
  omega_B/1 -> Cross Product/1

== system SimulationEnvManual/Plant/Drone/Moment Equation ==
  M : Inport
  Cross Product1 : matrix_library/Cross Product
  Integrator2 : Integrator
  Multiply2 : Gain  Gain=drone.I  Multiplication=Matrix(K*u)
  Multiply3 : Gain  Gain=(drone.I)^-1  Multiplication=Matrix(K*u)
  Sum1 : Sum  Inputs=+-
  omega_B : Outport
  wires:
  Cross Product1/1 -> Sum1/2
  M/1 -> Sum1/1
  Multiply2/1 -> Cross Product1/2
  Multiply3/1 -> Integrator2/1  "omega_BDot"
  Sum1/1 -> Multiply3/1
  Integrator2/1 -> Multiply2/1, Cross Product1/1, omega_B/1  "omega_B"

== matlab function SimulationEnvManual/Controller/MATLAB Function ==
  data: BIGL input; L output; psi input
function L = SelectLQR(BIGL, psi)

index = round(mod(180/pi*psi,360));

if index == 0 || index == 360
    index = 360;
end

L = BIGL(:,:,index);

== matlab function SimulationEnvManual/Subsystem/  ==
  data: phi input; R output; theta input; psi input
function R = B2B0(phi, theta, psi)

R = [cos(theta)*cos(psi),   sin(phi)*sin(theta)*cos(psi) - cos(phi)*sin(psi),   cos(phi)*sin(theta)*cos(psi)+sin(phi)*sin(psi);
     cos(theta)*sin(psi),   sin(phi)*sin(theta)*sin(psi) + cos(phi)*cos(psi),   cos(phi)*sin(theta)*sin(psi)-sin(phi)*cos(psi);
     -sin(theta)        ,   sin(phi)*cos(theta)                             ,   cos(phi)*cos(theta)                           ];

== matlab function SimulationEnvManual/Plant/Drone/R - from InitBody to Body ==
  data: phi input; R output; theta input; psi input
function R = B02B(phi, theta, psi)

R = [cos(theta)*cos(psi),   sin(phi)*sin(theta)*cos(psi) - cos(phi)*sin(psi),   cos(phi)*sin(theta)*cos(psi)+sin(phi)*sin(psi);
     cos(theta)*sin(psi),   sin(phi)*sin(theta)*sin(psi) + cos(phi)*cos(psi),   cos(phi)*sin(theta)*sin(psi)-sin(phi)*cos(psi);
     -sin(theta)        ,   sin(phi)*cos(theta)                             ,   cos(phi)*cos(theta)                           ]';

== matlab function SimulationEnvManual/Plant/Drone/Euler Kinematics/MATLAB Function ==
  data: p input; omega output; q input; r input; phi input; theta input
function omega = fcn(p,q,r, phi, theta)

% T = [1,     0           ,   sin(theta);
%      0,     cos(phi)    ,   -sin(phi)*cos(theta);
%      0,     sin(phi)    ,   cos(theta)*cos(phi)];

T_inv = [1,     tan(theta)*sin(phi)     ,   -tan(theta)*cos(phi);
         0,     cos(phi)                ,   sin(phi);
         0,     -sin(phi)/cos(theta)    ,  cos(phi)/cos(theta)];

omega = T_inv*[p;q;r];

== matlab function SimulationEnvManual/EKF/MATLAB Function ==
  data: muBar output; mu input; input input; Sigma input; SigmaBar output; g input; m input; I input; R input; fs input
function [muBar, SigmaBar] = prediction(mu, input, Sigma, g, m, I, R, fs)

% for different prediction model, change function name (predict,
% predictSimple)

[muBar, SigmaBar] = predict(mu, input, Sigma, g, m, I, R, fs);

== matlab function SimulationEnvManual/EKF/MATLAB Function1 ==
  data: SigmaBar input; K output; H input; Sigma output; Q input
function [K, Sigma] = calc_k_sigma(SigmaBar, H, Q)

[K, Sigma] = kalman_gain(SigmaBar, H, Q);

== matlab function SimulationEnvManual/EKF/MATLAB Function2 ==
  data: world input; muBar input; zBar output; H output
function [zBar, H] = predict_z(world, muBar)

[zBar, H] = predict_measurement(muBar, world);

== matlab function SimulationEnvManual/EKF/MATLAB Function3 ==
  data: muBar input; mu output; K input; zBar input; z input
function mu = update_mu(muBar, K, zBar, z)

%K=zeros(size(K)); % Uncomment to simulate without correction

mu = update(muBar, K, zBar, z);

== matlab function SimulationEnvManual/Generate Measurements/MATLAB Function ==
  data: xyp input; x output; world input; y output; z output
function [x,y,z]  = Meas2Pos(xyp, world)
Tb = world(1); hb = world(2); Lb = world(3); g = world(4); M = world(5); R = world(6); Pb = world(7);

x = xyp(1);
y = xyp(2);
z = -( Tb*( 1 - (xyp(3)/Pb)^( (R*Lb)/(g*M) ) ) / Lb + hb );

== matlab function SimulationEnvManual/Generate Measurements/Barometer/MATLAB Function ==
  data: Z input; std input; world input; P output
function P = fcn(Z, std, world)

Tb = world(1); hb = world(2); Lb = world(3); g = world(4); M = world(5); R = world(6); Pb = world(7);

P = Pb * ( (Tb-((-Z)-hb)*Lb) / Tb ) ^ (g*M/(R*Lb));
 
noise = std*randn;

P = P + noise;

%Z = Tb*( 1 - (P/Pb)^( (R*Lb)/(g*M) ) ) / Lb + hb;
end
